simulink model "Esercizio3_sim"  (R2022a)
settings: Solver=VariableStepAuto  StartTime=0.0  StopTime=2  RelTol=1e-3
values from neighbouring files (symbols this model uses):
  den = conv([ 1 1], [1/100 1])    [Esercizio3.m]    (also in myESE2.m)
  num = 10    [Esercizio3.m]    (also in myESE2.m)
undefined symbols (not defined in the file or in its folder): k, p, z
settings Model: Creator=chiar  LastModifiedBy=Stefano
settings SolverCC: AlgebraicLoopSolver=TrustRegion
settings DebuggingCC: UnconnectedInputMsg=warning  UnconnectedOutputMsg=warning  UnconnectedLineMsg=warning  SFMachineParentedDataDiag=warning
settings RTWCC: DLArmComputeVersion=19.05

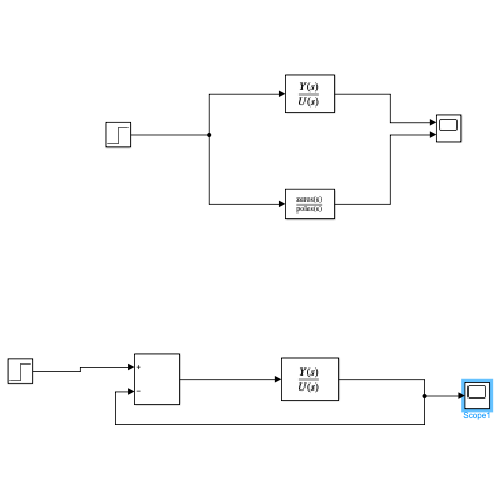
[thumbnail: Simulink's stored preview of the top-level diagram]
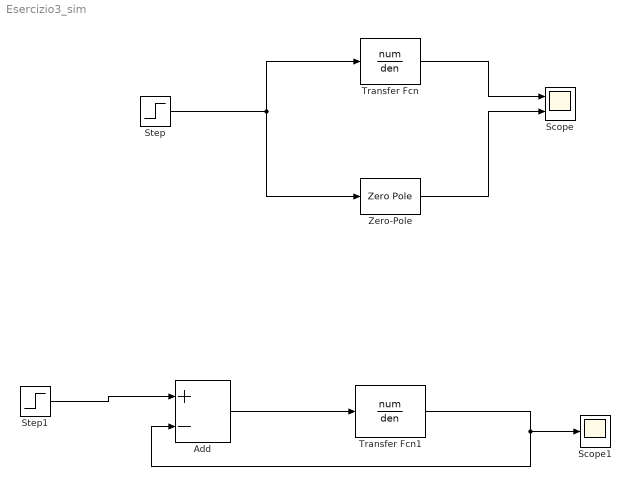
== system Esercizio3_sim ==
  Add : Sum  Inputs=+-
  Scope : Scope  NumInputPorts=2
  Scope1 : Scope
  Step : Step  SampleTime=0
  Step1 : Step  SampleTime=0
  Transfer Fcn : TransferFcn  Numerator=num  Denominator=den
  Transfer Fcn1 : TransferFcn  Numerator=num  Denominator=den
  Zero-Pole : ZeroPole  Zeros=z  Poles=p  Gain=k
  wires:
  Step/1 -> Transfer Fcn/1, Zero-Pole/1
  Transfer Fcn/1 -> Scope/1
  Zero-Pole/1 -> Scope/2
  Step1/1 -> Add/1
  Add/1 -> Transfer Fcn1/1
  Transfer Fcn1/1 -> Add/2, Scope1/1
